simulink model "MSAP_CV_bo"  (R2019b)
settings: Solver=ode4  StartTime=0.0  StopTime=2  FixedStep=1e-6  RelTol=1e-3
InitFcn:
  | % Paramètres (Test initial)
  | clc;
  | clear all;
  | 
  | Rs = 0.8;        % Résistance statorique
  | Ld = 1.1e-3;     % Inductance axe d
  | Lq = 1.32e-3;     % Inductance axe q
  | %Qf=1.5;        % Flux des aimants (Phi_f)
  | p = 2;           % Nombre de paires de pôles
  | J = 9.14e-2;     % Moment d'inertie
  | fr = 0.59e-4;     % Coefficient de frottement
  | 
  | 
  | 
  | 
  | 
  | 
  | Qf= 0.15;       % Flux des aimants (Phi_f)
libraries: powerlib x6, simulink x1
settings Model: Creator=x1 yoga  LastModifiedBy=x1 yoga

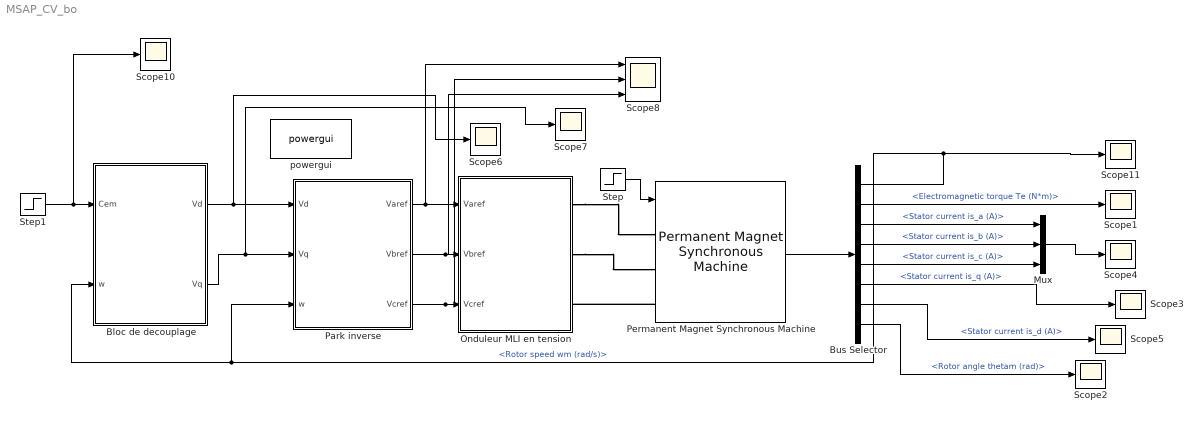
== system MSAP_CV_bo ==
  Bloc de decouplage : Subsystem
  Bus Selector : BusSelector  OutputSignals=Rotor speed wm (rad/s),Electromagnetic torque Te (N*m),Stator current is_a (A),Stator current is_b (A),Stator current is_c (A),Stator current is_q (A),Stator current is_d (A),Rotor angle thetam (rad)
  Mux : Mux  Inputs=3
  Onduleur MLI en tension : Subsystem
  Park inverse : Subsystem
  Permanent Magnet Synchronous Machine : powerlib/Machines/Permanent Magnet Synchronous Machine  NbPhases=3  FluxDistribution=Sinusoidal  RotorType=Salient-pole  MechanicalLoad=Torque Tm  PresetModel=No  ShowDetailedParameters=on  MeasurementBus=off  Resistance=0.8  Inductance=8.5e-3  dqInductances=[1.10e-3 1.32e-3]  La=0.000395  MachineConstant=Flux linkage established by magnets (V.s)  Flux=0.61  VoltageCst=221.2835  TorqueCst=1.83  Flat=120  Mechanical=[9.14e-2 0.59e-2 2 0]  PolePairs=4  InitialConditions=[0,0, 0,0]  InitialConditions5ph=[0 0 0 0 0 0]  RefAngle=Aligned with phase A axis (original Park)  IterativeDiscreteModel=Trapezoidal non iterative  TsBlock=-1  TsPowergui=0
  Scope{1..7,10..11} (9 alike) : Scope
  Scope8 : Scope  NumInputPorts=3
  Step : Step  Time=0.5  After=8  SampleTime=0
  Step1 : Step  Before=4  After=-4  SampleTime=0
  powergui : powerlib/powergui  Priority=1  SimulationMode=Continuous  SampleTime=50e-6  frequency=60  Iterations=50  frequencyindice=0  Pbase=100e6  ErrMax=1e-4  UnitsV=kV  UnitsW=MW  buscounter=0  FunctionMessages=off  echomessages=off  EnableUseOfTLC=off  CurrentSourceSwitches=off  DisableSnubberDevices=off  DisableRonSwitches=off  DisableVfSwitches=off  DisplayEquations=off  AutomaticDiscreteSolvers=off  SolverType=Tustin/Backward Euler (TBE)  Interpol=off  ExternalGateDelay=off  methode=off  Ts=100  x0status=blocks  SPID=on  SwTol=0  HookPort=off  NonlinearTolerance=1e-4  nMaxIteration=100  ContinueOnMaxIteration=off  RestoreLinks=warning  ResistiveCurrentMeasurement=off  Frange=[0:2:500]  Ylog=off  Xlog=on  ShowGrid=off  save=off  variable=ZData  structure=0  ZoomFFT=off  StartTime=0.0  cycles=1  DisplayStyle=1  fundamental=60  FreqAxis=off  MaxFrequency=1000  frequencyindicesteady=1  RmsSteady=1  display=off
      settings: SourceProductName=Simscape Electrical
  wires:
  Permanent Magnet Synchronous Machine/1 -> Bus Selector/1
  Bus Selector/7 -> Scope5/1  "<Stator current is_d (A)>"
  Mux/1 -> Scope4/1
  Bus Selector/8 -> Scope2/1  "<Rotor angle thetam (rad)>"
  Bus Selector/3 -> Mux/1  "<Stator current is_a (A)>"
  Bus Selector/6 -> Scope3/1  "<Stator current is_q (A)>"
  Bus Selector/2 -> Scope1/1  "<Electromagnetic torque Te (N*m)>"
  Bus Selector/4 -> Mux/2  "<Stator current is_b (A)>"
  Bus Selector/5 -> Mux/3  "<Stator current is_c (A)>"
  Bus Selector/1 -> Park inverse/3("w "), Bloc de decouplage/2(w), Scope11/1  "<Rotor speed wm (rad/s)>"
  Bloc de decouplage/1(Vd) -> Scope6/1, Park inverse/1(Vd)
  Bloc de decouplage/2(Vq) -> Scope7/1, Park inverse/2(Vq)
  Park inverse/1("Varef ") -> Onduleur MLI en tension/1(Varef), Scope8/1
  Park inverse/2("Vbref ") -> Scope8/3, Onduleur MLI en tension/2(Vbref)
  Park inverse/3("Vcref ") -> Scope8/2, Onduleur MLI en tension/3(Vcref)
  Step1/1 -> Scope10/1, Bloc de decouplage/1(Cem)
  Step/1 -> Permanent Magnet Synchronous Machine/1
  connections:
  Onduleur MLI en tension/RConn1 -- Permanent Magnet Synchronous Machine/LConn1
  Onduleur MLI en tension/RConn2 -- Permanent Magnet Synchronous Machine/LConn2
  Permanent Magnet Synchronous Machine/LConn3 -- Onduleur MLI en tension/RConn3

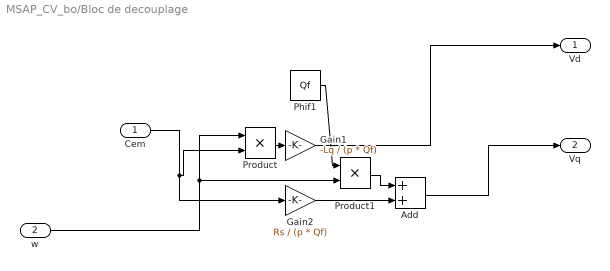
== system MSAP_CV_bo/Bloc de decouplage ==
  Cem : Inport
  w : Inport  Port=2
  Add : Sum
  Gain1 : Gain  Gain=-Lq / (p * Qf)
  Gain2 : Gain  Gain=Rs / (p * Qf)
  Phif1 : Constant  Value=Qf
  Product : Product
  Product1 : Product
  Vd : Outport
  Vq : Outport  Port=2
  wires:
  Add/1 -> Vq/1
  w/1 -> Product/1, Product1/2
  Gain1/1 -> Vd/1
  Cem/1 -> Gain2/1, Product/2
  Product/1 -> Gain1/1
  Gain2/1 -> Add/2
  Product1/1 -> Add/1
  Phif1/1 -> Product1/1

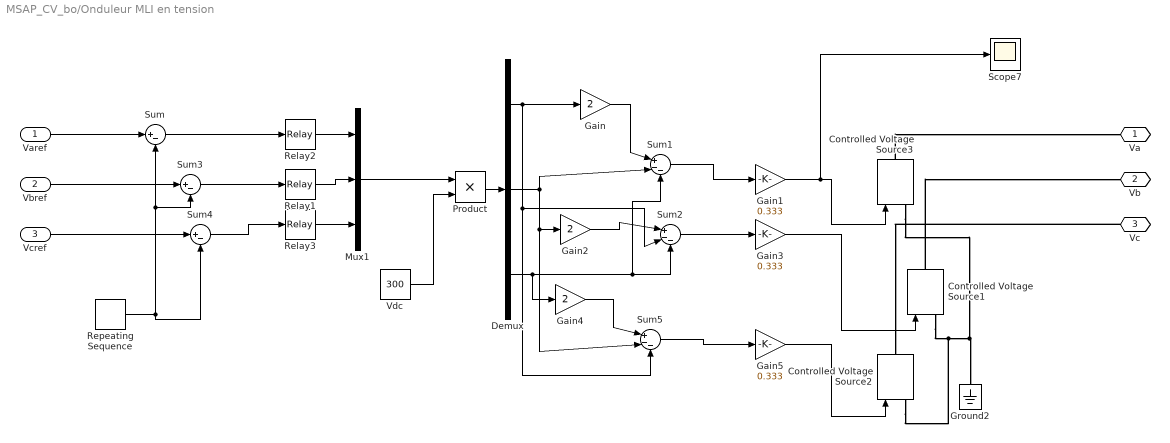
== system MSAP_CV_bo/Onduleur MLI en tension ==
  Varef : Inport
  Vbref : Inport  Port=2
  Vcref : Inport  Port=3
  Controlled Voltage Source1 : powerlib/Electrical Sources/Controlled Voltage Source  Initialize=on  Source_Type=AC  Amplitude=0  Phase=0  Frequency=0  Measurements=None
      settings: SourceProductName=Simscape Electrical
  Controlled Voltage Source2 : powerlib/Electrical Sources/Controlled Voltage Source  Initialize=on  Source_Type=AC  Amplitude=0  Phase=0  Frequency=0  Measurements=None
      settings: SourceProductName=Simscape Electrical
  Controlled Voltage Source3 : powerlib/Electrical Sources/Controlled Voltage Source  Initialize=on  Source_Type=AC  Amplitude=0  Phase=0  Frequency=0  Measurements=None
      settings: SourceProductName=Simscape Electrical
  Demux : Demux  Outputs=3
  Gain : Gain  Gain=2
  Gain1 : Gain  Gain=0.333
  Gain2 : Gain  Gain=2
  Gain3 : Gain  Gain=0.333
  Gain4 : Gain  Gain=2
  Gain5 : Gain  Gain=0.333
  Ground2 : powerlib/Elements/Ground  LConnTagsString=a
      settings: SourceProductName=Simscape Electrical
  Mux1 : Mux  Inputs=3
  Product : Product
  Relay1 : Relay
  Relay2 : Relay
  Relay3 : Relay
  Repeating Sequence : simulink/Sources/Repeating Sequence  rep_seq_t=[0 1/2 1]*(1/20000)  rep_seq_y="[-150  150  -150 ]*1"
  Scope7 : Scope
  Sum : Sum  Inputs=|+-
  Sum1 : Sum  Inputs=|+--
  Sum2 : Sum  Inputs=|+--
  Sum3 : Sum  Inputs=|+-
  Sum4 : Sum  Inputs=|+-
  Sum5 : Sum  Inputs=|+--
  "Vdc " : Constant  Value=300
  Va : PMIOPort  Side=Right
  Vb : PMIOPort  Port=2  Side=Right
  Vc : PMIOPort  Port=3  Side=Right
  wires:
  Sum2/1 -> Gain3/1
  Sum5/1 -> Gain5/1
  Varef/1 -> Sum/1
  Gain2/1 -> Sum2/1
  Sum4/1 -> Relay3/1
  Repeating Sequence/1 -> Sum4/2, Sum3/2, Sum/2
  Vbref/1 -> Sum3/1
  Sum/1 -> Relay2/1
  Sum3/1 -> Relay1/1
  Demux/2 -> Sum5/2, Gain2/1, Sum1/2
  Gain4/1 -> Sum5/1
  Demux/3 -> Gain4/1, Sum2/3, Sum1/3
  Relay2/1 -> Mux1/1
  Demux/1 -> Sum5/3, Sum2/2, Gain/1
  Vcref/1 -> Sum4/1
  Sum1/1 -> Gain1/1
  Gain/1 -> Sum1/1
  Relay3/1 -> Mux1/3
  "Vdc "/1 -> Product/2
  Mux1/1 -> Product/1
  Product/1 -> Demux/1
  Relay1/1 -> Mux1/2
  Gain1/1 -> Scope7/1, Controlled Voltage Source3/1
  Gain3/1 -> Controlled Voltage Source1/1
  Gain5/1 -> Controlled Voltage Source2/1
  connections:
  Controlled Voltage Source1/LConn1 -- Controlled Voltage Source2/LConn1 -- Controlled Voltage Source3/LConn1 -- Ground2/LConn1
  Controlled Voltage Source3/RConn1 -- Va/RConn1
  Vc/RConn1 -- Controlled Voltage Source2/RConn1
  Controlled Voltage Source1/RConn1 -- Vb/RConn1

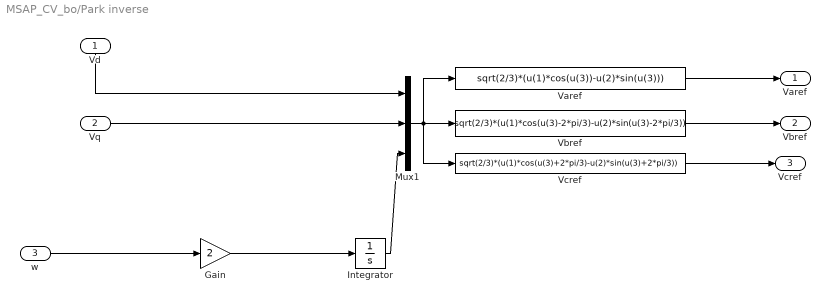
== system MSAP_CV_bo/Park inverse ==
  Vd : Inport
  Vq : Inport  Port=2
  "w " : Inport  Port=3
  Gain : Gain  Gain=2
  Integrator : Integrator
  Mux1 : Mux  Inputs=3
  Varef : Fcn  Expr=sqrt(2/3)*(u(1)*cos(u(3))-u(2)*sin(u(3)))
  Vbref : Fcn  Expr=sqrt(2/3)*(u(1)*cos(u(3)-2*pi/3)-u(2)*sin(u(3)-2*pi/3))
  Vcref : Fcn  Expr=sqrt(2/3)*(u(1)*cos(u(3)+2*pi/3)-u(2)*sin(u(3)+2*pi/3))
  "Varef " : Outport
  "Vbref " : Outport  Port=2
  "Vcref " : Outport  Port=3
  wires:
  Vcref/1 -> "Vcref "/1
  Integrator/1 -> Mux1/3
  Varef/1 -> "Varef "/1
  Vbref/1 -> "Vbref "/1
  Mux1/1 -> Vcref/1, Vbref/1, Varef/1
  "w "/1 -> Gain/1
  Vd/1 -> Mux1/1
  Vq/1 -> Mux1/2
  Gain/1 -> Integrator/1
